simulink model "Simulationsmodell_Diesel"  (R2020b)
settings: Solver=FixedStepAuto  StartTime=0.0  StopTime=simtime  FixedStep=1  RelTol=1e-3
undefined symbols (not defined in the file): c_d, c_r, converter_eff, eta_getriebe, fzBreite, fzBreiteInklSpiegel, fzHoehe, g, i_getriebe, i_mainreducer, kennfeld, lambda, luftdruck, M_bus, M_fahrgast, podesthoehe, R_Reifen, taupunkt, temperatur, torque_outputDivInput, tr_speed_ratio, tr_torque_ratio
settings Model: OrderedModelArguments=off  Creator=igyun  LastModifiedBy=user

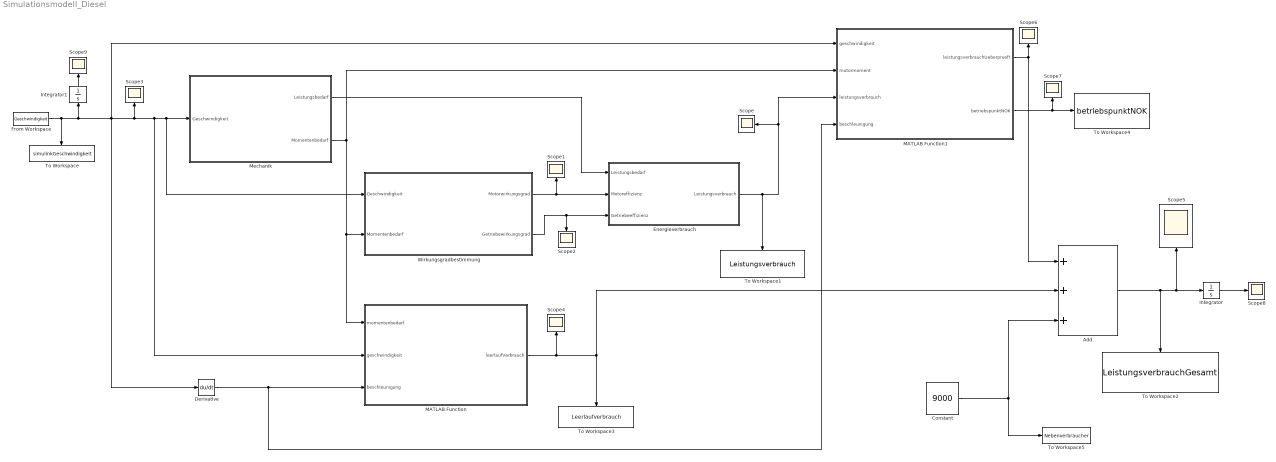
== system Simulationsmodell_Diesel ==
  Add : Sum  Inputs=+++
  Constant : Constant  Value=9000
  Derivative : Derivative
  Energieverbrauch : Subsystem
  From Workspace : FromWorkspace  VariableName=Geschwindigkeit
  Integrator : Integrator
  Integrator1 : Integrator
  MATLAB Function : MATLAB Function  TreatAsAtomicUnit=on
  MATLAB Function1 : MATLAB Function  TreatAsAtomicUnit=on
  Mechanik : Subsystem
  Scope{,1..9} (10 alike) : Scope
  To Workspace : ToWorkspace  VariableName=simulinkGeschwindigkeit  SaveFormat=Timeseries  SampleTime=-1
  To Workspace1 : ToWorkspace  VariableName=Leistungsverbrauch  SaveFormat=Timeseries  SampleTime=-1
  To Workspace2 : ToWorkspace  VariableName=LeistungsverbrauchGesamt  SaveFormat=Timeseries  SampleTime=-1
  To Workspace3 : ToWorkspace  VariableName=Leerlaufverbrauch  SaveFormat=Timeseries  SampleTime=-1
  To Workspace4 : ToWorkspace  VariableName=betriebspunktNOK  SaveFormat=Timeseries  SampleTime=-1
  To Workspace5 : ToWorkspace  VariableName=Nebenverbraucher  SaveFormat=Timeseries  SampleTime=-1
  Wirkungsgradbestimmung : Subsystem
  wires:
  Mechanik/1(Leistungsbedarf) -> Energieverbrauch/1(Leistungsbedarf)
  From Workspace/1 -> Wirkungsgradbestimmung/1(Geschwindigkeit), Mechanik/1(Geschwindigkeit), MATLAB Function/2(geschwindigkeit), Scope3/1, MATLAB Function1/1(geschwindigkeit), Derivative/1, Integrator1/1, To Workspace/1
  Mechanik/2(Momentenbedarf) -> MATLAB Function1/2(motormoment), MATLAB Function/1(momentenbedarf), Wirkungsgradbestimmung/2(Momentenbedarf)
  Wirkungsgradbestimmung/1(Motorwirkungsgrad) -> Scope1/1, Energieverbrauch/2(Motoreffizienz)
  Wirkungsgradbestimmung/2(Getriebewirkungsgrad) -> Energieverbrauch/3(Getriebeeffizienz), Scope2/1
  Energieverbrauch/1(Leistungsverbrauch) -> MATLAB Function1/3(leistungsverbrauch), Scope/1, To Workspace1/1
  Derivative/1 -> MATLAB Function/3(beschleunigung), MATLAB Function1/4(beschleunigung)
  MATLAB Function/1(leerlaufVerbrauch) -> To Workspace3/1, Add/2, Scope4/1
  Add/1 -> To Workspace2/1, Integrator/1, Scope5/1
  MATLAB Function1/1(leistungsverbrauchUeberprueft) -> Add/1, Scope6/1
  MATLAB Function1/2(betriebspunktNOK) -> To Workspace4/1, Scope7/1
  Integrator/1 -> Scope8/1
  Integrator1/1 -> Scope9/1
  Constant/1 -> To Workspace5/1, Add/3

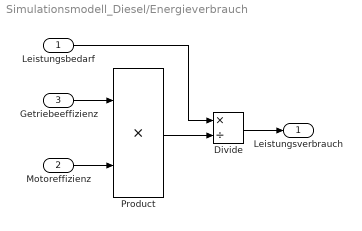
== system Simulationsmodell_Diesel/Energieverbrauch ==
  Leistungsbedarf : Inport
  Motoreffizienz : Inport  Port=2
  Getriebeeffizienz : Inport  Port=3
  Divide : Product  Inputs=*/
  Product : Product
  Leistungsverbrauch : Outport
  wires:
  Getriebeeffizienz/1 -> Product/1
  Motoreffizienz/1 -> Product/2
  Leistungsbedarf/1 -> Divide/1
  Product/1 -> Divide/2
  Divide/1 -> Leistungsverbrauch/1

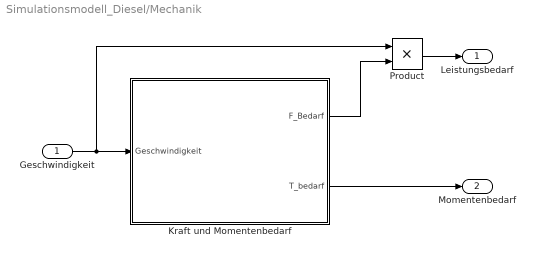
== system Simulationsmodell_Diesel/Mechanik ==
  Geschwindigkeit : Inport
  Kraft und Momentenbedarf : Subsystem
  Product : Product
  Leistungsbedarf : Outport
  Momentenbedarf : Outport  Port=2
  wires:
  Product/1 -> Leistungsbedarf/1
  Kraft und Momentenbedarf/1(F_Bedarf) -> Product/2
  Geschwindigkeit/1 -> Kraft und Momentenbedarf/1(Geschwindigkeit), Product/1
  Kraft und Momentenbedarf/2(T_bedarf) -> Momentenbedarf/1

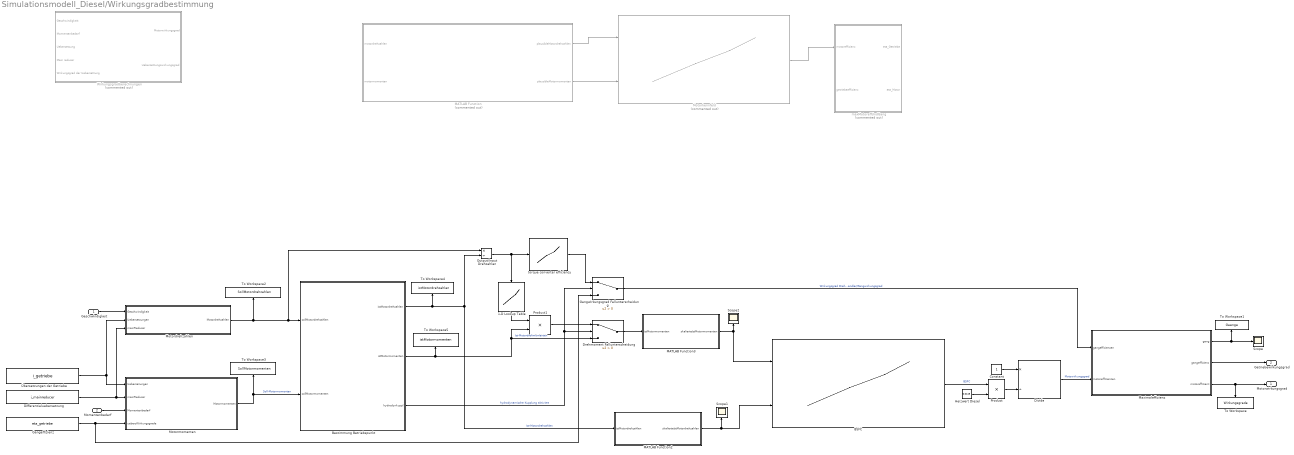
== system Simulationsmodell_Diesel/Wirkungsgradbestimmung ==
  Geschwindigkeit : Inport
  Momentenbedarf : Inport  Port=2
  1-D Lookup Table : Lookup_n-D  NumberOfTableDimensions=1  BreakpointsForDimension1=tr_speed_ratio  Table=tr_torque_ratio  InternalRulePriority=Speed  RndMeth=Simplest  InputSameDT=on
  BSFC : Lookup_n-D  BreakpointsForDimension1=[1:91]  BreakpointsForDimension2=[1:166]  Table=kennfeld  InternalRulePriority=Speed  RndMeth=Simplest  InputSameDT=on
      settings: InputPortMap=u0,u1
  Bestimmung Betriebspunkt : MATLAB Function  TreatAsAtomicUnit=on
  Constant : Constant
  Differentialuebersetzung : Constant  Value=i_mainreducer
  Divide : Product  Inputs=*/
  Drehmoment Fallunterscheidung : Switch  Criteria=u2 > Threshold
  Gangeffizienz : Constant  Value=eta_getriebe
  Gangwirkungsgrad Fallunterscheidung : Switch  Criteria=u2 > Threshold
  Heizwert Diesel : Constant  Value=0.0119
  MATLAB Function : MATLAB Function  Commented=on  TreatAsAtomicUnit=on
  MATLAB Function2 : MATLAB Function  TreatAsAtomicUnit=on
  MATLAB Function3 : MATLAB Function  TreatAsAtomicUnit=on
  Maximaleffizienz : MATLAB Function  TreatAsAtomicUnit=on
  Motordrehzahlen : Subsystem
  Motorkennfeld : Lookup_n-D  Commented=on  BreakpointsForDimension1=[1:86]  BreakpointsForDimension2=[1:251]  Table=kennfeld  InternalRulePriority=Speed  RndMeth=Simplest  InputSameDT=on
      settings: InputPortMap=u0,u1
  Motormomenten : Subsystem
  Output/Input Drehzahlen : Product  Inputs=*/
  Product : Product
  Product1 : Product
  Scope : Scope
  Scope1 : Scope
  Scope2 : Scope
  To Workspace : ToWorkspace  VariableName=Wirkungsgrade  SaveFormat=Timeseries  SampleTime=-1
  To Workspace1 : ToWorkspace  VariableName=Gaenge  SaveFormat=Timeseries  SampleTime=-1
  To Workspace2 : ToWorkspace  VariableName=SollMotordrehzahlen  SaveFormat=Timeseries  SampleTime=-1
  To Workspace3 : ToWorkspace  VariableName=SollMotormomenten  SaveFormat=Timeseries  SampleTime=-1
  To Workspace4 : ToWorkspace  VariableName=istMotordrehzahlen  SaveFormat=Timeseries  SampleTime=-1
  To Workspace5 : ToWorkspace  VariableName=istMotormomenten  SaveFormat=Timeseries  SampleTime=-1
  Wirkungsgradberechnungen : Subsystem  Commented=on  TreatAsAtomicUnit=on
  maxMotoreffUndGang : MATLAB Function  Commented=on  TreatAsAtomicUnit=on
  torque converter efficiency : Lookup_n-D  NumberOfTableDimensions=1  BreakpointsForDimension1=torque_outputDivInput  Table=converter_eff  InternalRulePriority=Speed  RndMeth=Simplest  InputSameDT=on
  Übersetzungen der Getriebe : Constant  Value=i_getriebe
  Motorwirkungsgrad : Outport
  Getriebewirkungsgrad : Outport  Port=2
  wires:
  Übersetzungen der Getriebe/1 -> Motormomenten/1(Uebersezungen), Motordrehzahlen/2(Uebersetzungen)
  Differentialuebersetzung/1 -> Motordrehzahlen/3(mainReducer), Motormomenten/2(mainReducer)
  Momentenbedarf/1 -> Motormomenten/3(Momentenbedarf)
  Gangeffizienz/1 -> Gangwirkungsgrad Fallunterscheidung/3, Motormomenten/4(uebersWirkungsgrade)
  MATLAB Function/1(plausibleMotordrehzahlen) -> Motorkennfeld/1
  MATLAB Function/2(plausibleMotormomenten) -> Motorkennfeld/2
  Motorkennfeld/1 -> maxMotoreffUndGang/1(motoreffizienz)
  Motordrehzahlen/1(Motordrehzahlen) -> To Workspace2/1, Output/Input Drehzahlen/1, Bestimmung Betriebspunkt/1(sollMotordrehzahlen)
  Motormomenten/1(Motormomenten) -> Bestimmung Betriebspunkt/2(sollMotormomenten), To Workspace3/1  "Soll-Motormomenten"
  Bestimmung Betriebspunkt/1(istMotordrehzahlen) -> MATLAB Function2/1(istMotordrehzahlen), Output/Input Drehzahlen/2, To Workspace4/1  "Ist-Motordrehzahlen"
  Output/Input Drehzahlen/1 -> 1-D Lookup Table/1, torque converter efficiency/1
  torque converter efficiency/1 -> Gangwirkungsgrad Fallunterscheidung/1
  Bestimmung Betriebspunkt/2(istMotormomenten) -> Product1/2, Drehmoment Fallunterscheidung/3, To Workspace5/1  "Ist-Motordrehmomenten"
  Bestimmung Betriebspunkt/3(hydrodynkuppl) -> Gangwirkungsgrad Fallunterscheidung/2, Drehmoment Fallunterscheidung/2  "hydrodynamische Kupplung aktiviert"
  Gangwirkungsgrad Fallunterscheidung/1 -> Maximaleffizienz/1(gangeffizienzen)  "Wirkungsgrad Drehmomentwandler/Gangwirkungsgrad"
  Maximaleffizienz/2(gangeffizienz) -> Getriebewirkungsgrad/1
  Maximaleffizienz/3(motoreffizienz) -> Motorwirkungsgrad/1, To Workspace/1
  Maximaleffizienz/1(gang) -> To Workspace1/1, Scope/1
  BSFC/1 -> Product/1  "BSFC"
  Constant/1 -> Divide/1
  Divide/1 -> Maximaleffizienz/2(motoreffizienzen)  "Motowirkungsgrad"
  Heizwert Diesel/1 -> Product/2
  Product/1 -> Divide/2
  1-D Lookup Table/1 -> Product1/1
  Product1/1 -> Drehmoment Fallunterscheidung/1
  Drehmoment Fallunterscheidung/1 -> MATLAB Function3/1(istMotormomenten)
  Geschwindigkeit/1 -> Motordrehzahlen/1(Geschwindigkeit)
  MATLAB Function2/1(skalierteIstMotordrehzahlen) -> BSFC/2, Scope1/1
  MATLAB Function3/1(skalierteIstMotormomenten) -> BSFC/1, Scope2/1

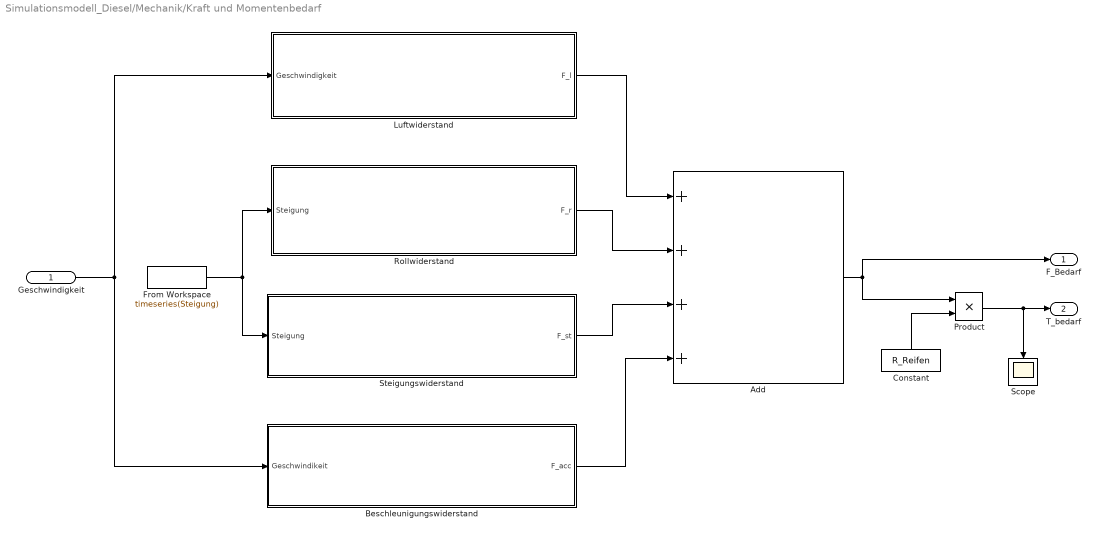
== system Simulationsmodell_Diesel/Mechanik/Kraft und Momentenbedarf ==
  Geschwindigkeit : Inport
  Add : Sum  Inputs=++++
  Beschleunigungswiderstand : Subsystem
  Constant : Constant  Value=R_Reifen
  From Workspace : FromWorkspace  VariableName=timeseries(Steigung)
  Luftwiderstand : Subsystem
  Product : Product
  Rollwiderstand : Subsystem
  Scope : Scope
  Steigungswiderstand : Subsystem
  F_Bedarf : Outport
  T_bedarf : Outport  Port=2
  wires:
  Geschwindigkeit/1 -> Beschleunigungswiderstand/1(Geschwindikeit), Luftwiderstand/1(Geschwindigkeit)
  Luftwiderstand/1(F_l) -> Add/1
  Beschleunigungswiderstand/1(F_acc) -> Add/4
  Rollwiderstand/1(F_r) -> Add/2
  Steigungswiderstand/1(F_st) -> Add/3
  Add/1 -> Product/1, F_Bedarf/1
  Constant/1 -> Product/2
  Product/1 -> T_bedarf/1, Scope/1
  From Workspace/1 -> Steigungswiderstand/1(Steigung), Rollwiderstand/1(Steigung)

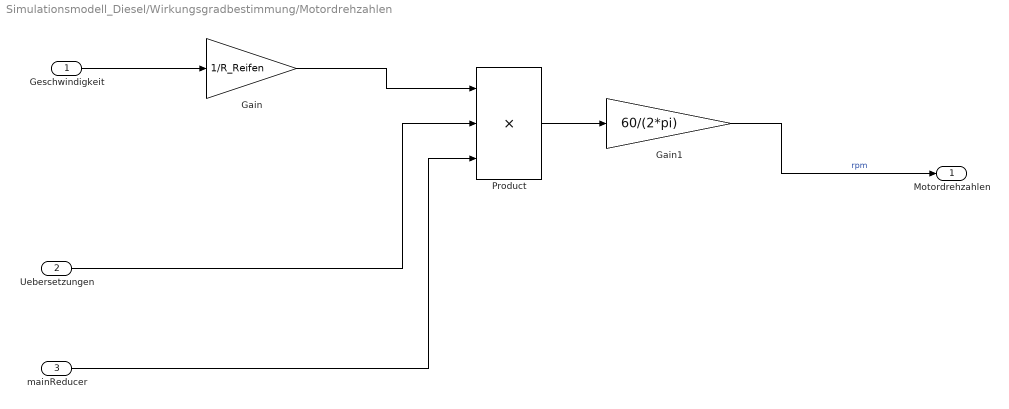
== system Simulationsmodell_Diesel/Wirkungsgradbestimmung/Motordrehzahlen ==
  Geschwindigkeit : Inport
  Uebersetzungen : Inport  Port=2
  mainReducer : Inport  Port=3
  Gain : Gain  Gain=1/R_Reifen
  Gain1 : Gain  Gain=60/(2*pi)
  Product : Product  Inputs=3
  Motordrehzahlen : Outport
  wires:
  Geschwindigkeit/1 -> Gain/1
  Product/1 -> Gain1/1
  Uebersetzungen/1 -> Product/2
  Gain/1 -> Product/1
  mainReducer/1 -> Product/3
  Gain1/1 -> Motordrehzahlen/1  "rpm"

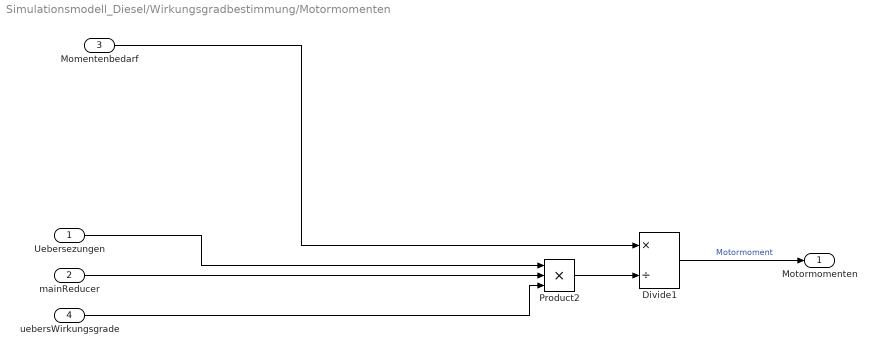
== system Simulationsmodell_Diesel/Wirkungsgradbestimmung/Motormomenten ==
  Uebersezungen : Inport
  mainReducer : Inport  Port=2
  Momentenbedarf : Inport  Port=3
  uebersWirkungsgrade : Inport  Port=4
  Divide1 : Product  Inputs=*/
  Product2 : Product  Inputs=3
  Motormomenten : Outport
  wires:
  uebersWirkungsgrade/1 -> Product2/3
  mainReducer/1 -> Product2/2
  Product2/1 -> Divide1/2
  Momentenbedarf/1 -> Divide1/1
  Uebersezungen/1 -> Product2/1
  Divide1/1 -> Motormomenten/1  "Motormoment"

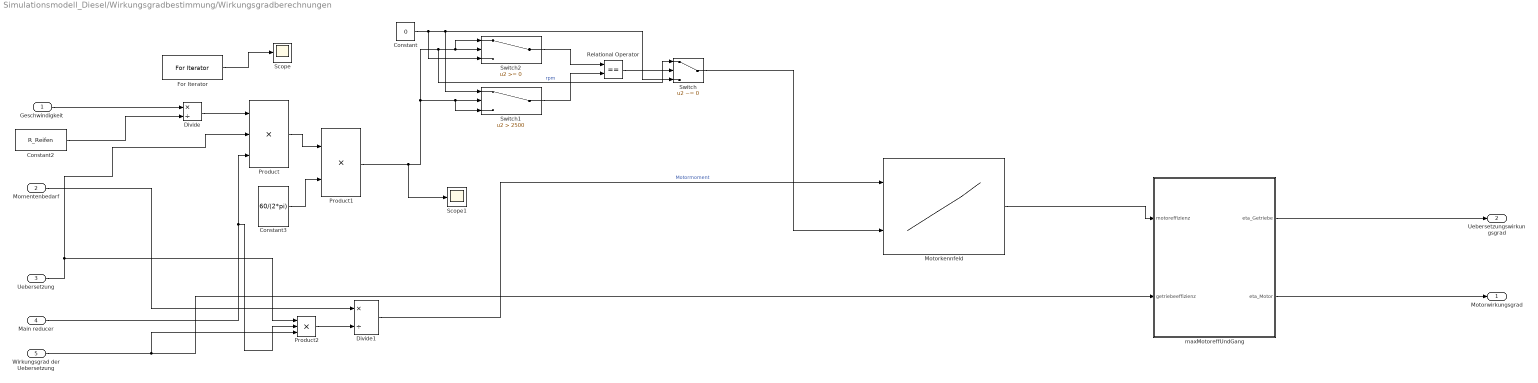
== system Simulationsmodell_Diesel/Wirkungsgradbestimmung/Wirkungsgradberechnungen ==
  Geschwindigkeit : Inport
  Momentenbedarf : Inport  Port=2
  Uebersetzung : Inport  Port=3
  Main reducer : Inport  Port=4
  Wirkungsgrad der Uebersetzung : Inport  Port=5
  Constant : Constant  Value=0
  Constant2 : Constant  Value=R_Reifen
  Constant3 : Constant  Value=60/(2*pi)
  Divide : Product  Inputs=*/
  Divide1 : Product  Inputs=*/
  For Iterator : ForIterator  IterationLimit=4
  Motorkennfeld : Lookup_n-D  BreakpointsForDimension1=[1:86]  BreakpointsForDimension2=[1:251]  Table=kennfeld  InternalRulePriority=Speed  RndMeth=Simplest  InputSameDT=on
      settings: InputPortMap=u0,u1
  Product : Product  Inputs=3
  Product1 : Product
  Product2 : Product  Inputs=3
  Relational Operator : RelationalOperator  Operator===  OutDataTypeStr=boolean  RndMeth=Simplest
  Scope : Scope
  Scope1 : Scope
  Switch : Switch  Criteria=u2 ~= 0  Threshold=1
  Switch1 : Switch  Criteria=u2 > Threshold  Threshold=2500
  Switch2 : Switch
  maxMotoreffUndGang : MATLAB Function  TreatAsAtomicUnit=on
  Motorwirkungsgrad : Outport
  Uebersetzungswirkungsgrad : Outport  Port=2
  wires:
  Constant3/1 -> Product1/2
  Product/1 -> Product1/1
  Constant2/1 -> Divide/2
  Geschwindigkeit/1 -> Divide/1
  Divide/1 -> Product/1
  Wirkungsgrad der Uebersetzung/1 -> maxMotoreffUndGang/2(getriebeeffizienz), Product2/3
  Main reducer/1 -> Product2/2, Product/3
  Uebersetzung/1 -> Product/2, Product2/1
  Product2/1 -> Divide1/2
  Momentenbedarf/1 -> Divide1/1
  Divide1/1 -> Motorkennfeld/1  "Motormoment"
  Motorkennfeld/1 -> maxMotoreffUndGang/1(motoreffizienz)
  maxMotoreffUndGang/1(eta_Getriebe) -> Uebersetzungswirkungsgrad/1
  maxMotoreffUndGang/2(eta_Motor) -> Motorwirkungsgrad/1
  For Iterator/1 -> Scope/1
  Switch2/1 -> Relational Operator/1
  Switch1/1 -> Relational Operator/2
  Constant/1 -> Switch2/3, Switch1/1, Switch/3
  Switch/1 -> Motorkennfeld/2
  Relational Operator/1 -> Switch/2
  Product1/1 -> Scope1/1, Switch1/3, Switch1/2, Switch/1, Switch2/1, Switch2/2  "rpm"

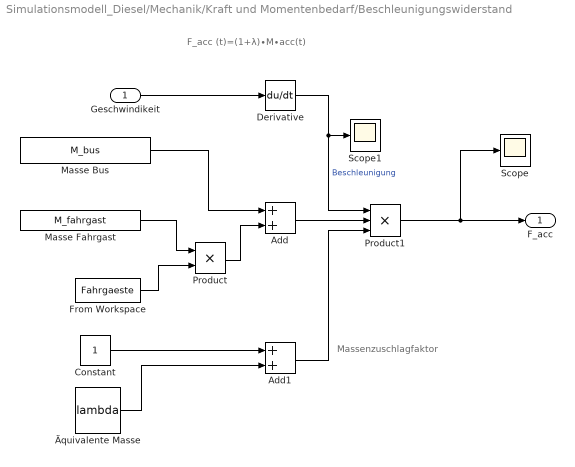
== system Simulationsmodell_Diesel/Mechanik/Kraft und Momentenbedarf/Beschleunigungswiderstand ==
  note: Massenzuschlagfaktor
  note: F_acc (t)=(1+λ)∙M∙acc(t)
  Geschwindikeit : Inport
  Add : Sum
  Add1 : Sum
  Constant : Constant
  Derivative : Derivative
  From Workspace : FromWorkspace  VariableName=Fahrgaeste
  Masse Bus : Constant  Value=M_bus
  Masse Fahrgast : Constant  Value=M_fahrgast
  Product : Product
  Product1 : Product  Inputs=3
  Scope : Scope
  Scope1 : Scope
  Äquivalente Masse : Constant  Value=lambda
  F_acc : Outport
  wires:
  Geschwindikeit/1 -> Derivative/1
  Masse Fahrgast/1 -> Product/1
  From Workspace/1 -> Product/2
  Masse Bus/1 -> Add/1
  Product/1 -> Add/2
  Constant/1 -> Add1/1
  Äquivalente Masse/1 -> Add1/2
  Derivative/1 -> Product1/1, Scope1/1  "Beschleunigung"
  Add/1 -> Product1/2
  Add1/1 -> Product1/3
  Product1/1 -> Scope/1, F_acc/1

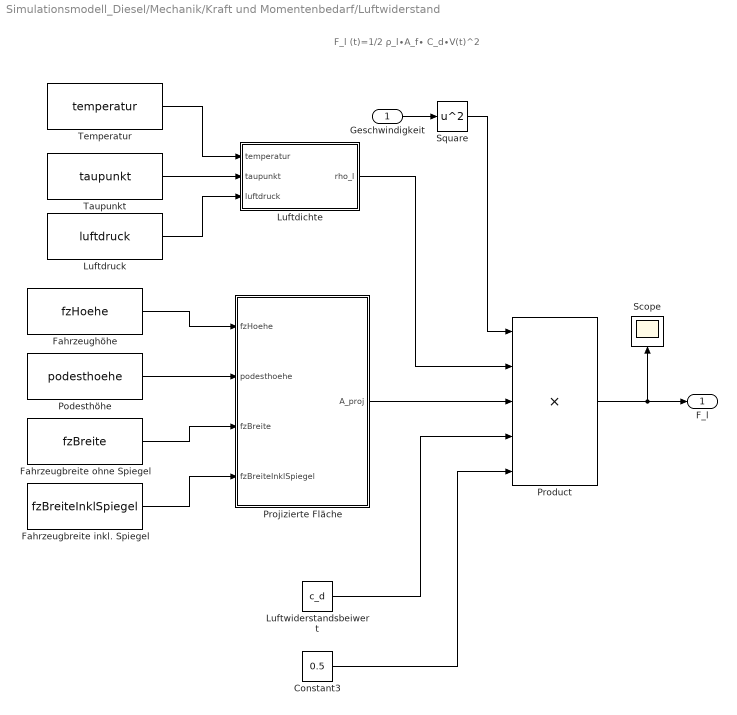
== system Simulationsmodell_Diesel/Mechanik/Kraft und Momentenbedarf/Luftwiderstand ==
  note: F_l (t)=1/2 ρ_l∙A_f∙ C_d∙V(t)^2
  Geschwindigkeit : Inport
  Constant3 : Constant  Value=0.5
  Fahrzeugbreite inkl. Spiegel : Constant  Value=fzBreiteInklSpiegel
  Fahrzeugbreite ohne Spiegel : Constant  Value=fzBreite
  Fahrzeughöhe : Constant  Value=fzHoehe
  Luftdichte : MATLAB Function  TreatAsAtomicUnit=on
  Luftdruck : Constant  Value=luftdruck
  Luftwiderstandsbeiwert : Constant  Value=c_d
  Podesthöhe : Constant  Value=podesthoehe
  Product : Product  Inputs=5
  Projizierte Fläche : MATLAB Function  TreatAsAtomicUnit=on
  Scope : Scope
  Square : Math  Operator=square  SaturateOnIntegerOverflow=on
  Taupunkt : Constant  Value=taupunkt
  Temperatur : Constant  Value=temperatur
  F_l : Outport
  wires:
  Geschwindigkeit/1 -> Square/1
  Square/1 -> Product/1
  Luftdichte/1(rho_l) -> Product/2
  Projizierte Fläche/1(A_proj) -> Product/3
  Luftwiderstandsbeiwert/1 -> Product/4
  Constant3/1 -> Product/5
  Product/1 -> F_l/1, Scope/1
  Temperatur/1 -> Luftdichte/1(temperatur)
  Taupunkt/1 -> Luftdichte/2(taupunkt)
  Luftdruck/1 -> Luftdichte/3(luftdruck)
  Fahrzeugbreite inkl. Spiegel/1 -> Projizierte Fläche/4(fzBreiteInklSpiegel)
  Fahrzeugbreite ohne Spiegel/1 -> Projizierte Fläche/3(fzBreite)
  Podesthöhe/1 -> Projizierte Fläche/2(podesthoehe)
  Fahrzeughöhe/1 -> Projizierte Fläche/1(fzHoehe)

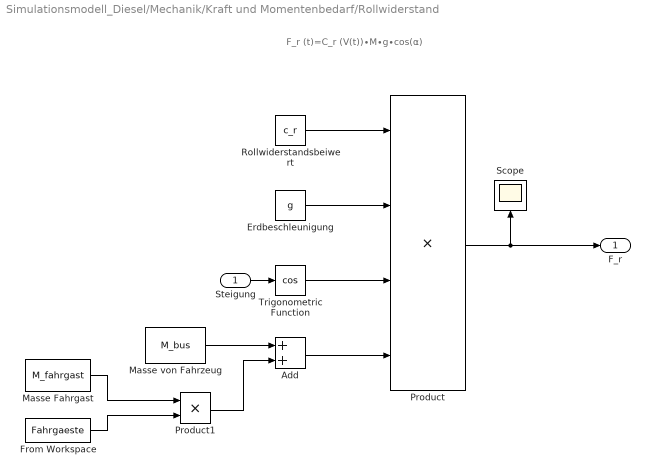
== system Simulationsmodell_Diesel/Mechanik/Kraft und Momentenbedarf/Rollwiderstand ==
  note: F_r (t)=C_r (V(t))∙M∙g∙cos⁡(α)
  Steigung : Inport
  Add : Sum
  Erdbeschleunigung : Constant  Value=g
  From Workspace : FromWorkspace  VariableName=Fahrgaeste
  Masse Fahrgast : Constant  Value=M_fahrgast
  Masse von Fahrzeug : Constant  Value=M_bus
  Product : Product  Inputs=4
  Product1 : Product
  Rollwiderstandsbeiwert : Constant  Value=c_r
  Scope : Scope
  Trigonometric Function : Trigonometry  Operator=cos
  F_r : Outport
  wires:
  Masse von Fahrzeug/1 -> Add/1
  Steigung/1 -> Trigonometric Function/1
  Add/1 -> Product/4
  Trigonometric Function/1 -> Product/3
  Erdbeschleunigung/1 -> Product/2
  Rollwiderstandsbeiwert/1 -> Product/1
  Product/1 -> F_r/1, Scope/1
  Masse Fahrgast/1 -> Product1/1
  From Workspace/1 -> Product1/2
  Product1/1 -> Add/2

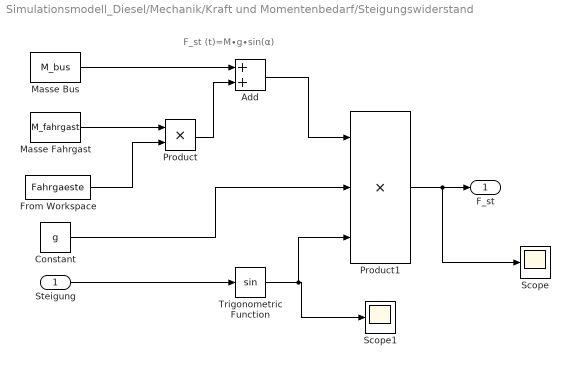
== system Simulationsmodell_Diesel/Mechanik/Kraft und Momentenbedarf/Steigungswiderstand ==
  note: F_st (t)=M∙g∙sin⁡(α)
  Steigung : Inport
  Add : Sum
  Constant : Constant  Value=g
  From Workspace : FromWorkspace  VariableName=Fahrgaeste
  Masse Bus : Constant  Value=M_bus
  Masse Fahrgast : Constant  Value=M_fahrgast
  Product : Product
  Product1 : Product  Inputs=3
  Scope : Scope
  Scope1 : Scope
  Trigonometric Function : Trigonometry
  F_st : Outport
  wires:
  Masse Fahrgast/1 -> Product/1
  From Workspace/1 -> Product/2
  Masse Bus/1 -> Add/1
  Product/1 -> Add/2
  Steigung/1 -> Trigonometric Function/1
  Add/1 -> Product1/1
  Trigonometric Function/1 -> Product1/3, Scope1/1
  Product1/1 -> Scope/1, F_st/1
  Constant/1 -> Product1/2

== matlab function Simulationsmodell_Diesel/MATLAB Function1 ==
  data: geschwindigkeit input; motormoment input; leistungsverbrauch input; leistungsverbrauchUeberprueft output; beschleunigung input; betriebspunktNOK output
function [leistungsverbrauchUeberprueft, betriebspunktNOK] = ueberpruefeNaN(geschwindigkeit, motormoment, leistungsverbrauch, beschleunigung)

    if isnan(leistungsverbrauch)
        if (geschwindigkeit == 0 && beschleunigung == 0) || motormoment <= 0
            leistungsverbrauchUeberprueft = 0;
            betriebspunktNOK = 0;
        else
            betriebspunktNOK = 1;
            leistungsverbrauchUeberprueft = 0;
        end
    else
        betriebspunktNOK = 0;
        leistungsverbrauchUeberprueft = leistungsverbrauch;
    end
        


end

== matlab function Simulationsmodell_Diesel/Mechanik/Kraft und Momentenbedarf/Luftwiderstand/Projizierte Fläche ==
  data: fzHoehe input; A_proj output; podesthoehe input; fzBreite input; fzBreiteInklSpiegel input
function A_proj = projflaeche(fzHoehe, podesthoehe, fzBreite, fzBreiteInklSpiegel)

    %Eingabe in Maske: mm
    
    A_proj1 = (fzHoehe-podesthoehe)*fzBreite;
    
    %Spiegelhöhe
    spiegelHoehe = 400;
    A_proj2 = (fzBreiteInklSpiegel-fzBreite)*spiegelHoehe;
    
    A_proj = A_proj1 + A_proj2;
    
    %Umrechung mm^2 in m^2;
    
    A_proj = A_proj * 10^-6;
    
end

== matlab function Simulationsmodell_Diesel/Mechanik/Kraft und Momentenbedarf/Luftwiderstand/Luftdichte ==
  data: temperatur input; rho_l output; taupunkt input; luftdruck input
function rho_l = luftdichte(temperatur, taupunkt, luftdruck)

%Für Werte: https://kachelmannwetter.com/site/auswahl

%Einheiten bei der Eingabemaske:
%Druck: hPa
%Temperatur: Celsius

%Temperaturumrechnung
temperatur = temperatur + 273.15;



%Konstanten aus https://www.gribble.org/cycling/air_density.html
c0 = 0.99999683;
c1 = -0.90826951e-2;
c2 = 0.78736169e-4;
c3 = -0.61117958e-6;
c4 = 0.43884187e-8;
c5 = -0.29883885e-10;
c6 = 0.21874425e-12;
c7 = -0.17892321e-14;
c8 = 0.11112018e-16;
c9 = -0.30994571e-19;

e_so = 6.1078;

R_v = 461.4964;
R_d=287.0531;

%Druck bei Sättigungstemperatur
p_taupunkt = c0 + taupunkt *(c1 + taupunkt*(c2 + taupunkt*(c3 + taupunkt*(c4 + taupunkt*(c5 + taupunkt*(c6 + taupunkt*(c7 + taupunkt*(c8 + taupunkt*(c9) ) ) ) ) ) ) ));

%Sättigungsdruck von Dampf
E_s = e_so./p_taupunkt.^8;
P_v = E_s;

%Luftdruck bei trockener Luft
P_d = luftdruck - P_v;

%Luftdichte in kg/m^3
rho_l =  (P_d*100 / (R_d * temperatur)) + (P_v*100 / (R_v * temperatur));
%Umrechnungsfaktor 100 von mbar(hPa) zu Pa
end

== matlab function Simulationsmodell_Diesel/Wirkungsgradbestimmung/MATLAB Function ==
  data: motordrehzahlen input; plausibleMotordrehzahlen output; motormomenten input; plausibleMotormomenten output
function [plausibleMotordrehzahlen, plausibleMotormomenten] = ueberpruefenDrehzahlDrehmoment(motordrehzahlen, motormomenten)
    %Vorerzeugen der Vektoren mit plausiblen Daten
    plausibleMotordrehzahlen = zeros(4,1);
    plausibleMotormomenten = zeros(4,1);
    for j = 1:4 %4 Gänge => 4 drehzahlen bzw. momenten
        if motordrehzahlen(j)<=2500 && motordrehzahlen(j)>=800 && motormomenten(j)>=0 && motormomenten(j)<=1200
            %Wenn die Bedingungen erfüllt sind, ist der Betriebspunkt
            %erreichbar
            plausibleMotordrehzahlen(j,1)=motordrehzahlen(j);
            plausibleMotormomenten(j,1)=motormomenten(j);
        else
            plausibleMotordrehzahlen(j,1)=0;
            plausibleMotormomenten(j,1)=0;
        end
    end
end

== matlab function Simulationsmodell_Diesel/Wirkungsgradbestimmung/Wirkungsgradberechnungen/maxMotoreffUndGang ==
  data: motoreffizienz input; eta_Getriebe output; getriebeeffizienz input; eta_Motor output
function [eta_Getriebe, eta_Motor] = wirkungsgradAuswahl(motoreffizienz, getriebeeffizienz)

for j = 2:length(motoreffizienz)
    if motoreffizienz(j)>motoreffizienz(j-1)
        index = j;
    else
        index = j-1;
    end
end
eta_Getriebe = getriebeeffizienz(index);
eta_Motor = motoreffizienz(index);

== matlab function Simulationsmodell_Diesel/Wirkungsgradbestimmung/maxMotoreffUndGang ==
  data: motoreffizienz input; eta_Getriebe output; getriebeeffizienz input; eta_Motor output
function [eta_Getriebe, eta_Motor] = wirkungsgradAuswahl(motoreffizienz, getriebeeffizienz)

for j = 2:length(motoreffizienz)
    if motoreffizienz(j)>motoreffizienz(j-1)
        index = j;
    else
        index = j-1;
    end
end
eta_Getriebe = getriebeeffizienz(index);
eta_Motor = motoreffizienz(index);

== matlab function Simulationsmodell_Diesel/Wirkungsgradbestimmung/Bestimmung Betriebspunkt ==
  data: sollMotordrehzahlen input; istMotordrehzahlen output; istMotormomenten output; hydrodynkuppl output; sollMotormomenten input
function [istMotordrehzahlen, istMotormomenten, hydrodynkuppl]  = betriebspunktBestimmungen(sollMotordrehzahlen, sollMotormomenten)
    
    %Mindestdrehzahlbestimmung 
    
    if sollMotordrehzahlen(1) < 800
        istMotordrehzahlen = zeros(length(sollMotordrehzahlen),1);
        %Für den Fall, dass sogar erster Gang die notwendige
        %Motordrehzahl nicht erreichen kann
        %Annahme: Minimaldrehzahl = 800 rpm
        
        istMotordrehzahlen(1) = 800; 
        
        %Hilfsvariable (es handelt sich um eine hydrodynamische Kupplung)
        hydrodynkuppl = 1;
        
        %Die restlichen Motordrehzahlen als NaN definieren
        
        istMotordrehzahlen(2) = NaN;
        istMotordrehzahlen(3) = NaN;
        istMotordrehzahlen(4) = NaN;
    else
        %Die notwendige Drehzahl wird mindestens von 1. Gang erreicht =>
        %keine hydrodynamische Kupplung notwendig
        hydrodynkuppl = 0;
        
        %Vorerzeugung der Größe des Vektors
        
        istMotordrehzahlen=zeros(length(sollMotordrehzahlen),1);
        
        %Überprüfen ob die Gänge im zul. Bereich liegen

        for ii = 1:length(sollMotordrehzahlen)
            if sollMotordrehzahlen(ii) >= 800 && sollMotordrehzahlen(ii) <= 2500
                %Zuvor berechnete Werte (soll) liegen im zul. Bereich =>
                %ist=soll
                istMotordrehzahlen(ii)=sollMotordrehzahlen(ii);
            else
                istMotordrehzahlen(ii) = NaN;
            end
        end
    end
    
    %zul. Drehmomente
    istMotormomenten = zeros(length(sollMotormomenten),1);
    
    for ii = 1:length(sollMotormomenten)
        
        %Definition der Obergrenze
        if sollMotormomenten(ii) >= 0 && sollMotormomenten(ii) <= 1200
            istMotormomenten(ii) = sollMotormomenten(ii);
        else
            istMotormomenten(ii) = NaN;
        end
        
    end


    
end

== matlab function Simulationsmodell_Diesel/Wirkungsgradbestimmung/Maximaleffizienz ==
  data: gang output; gangeffizienzen input; motoreffizienzen input; gangeffizienz output; motoreffizienz output
function [gang, gangeffizienz, motoreffizienz]= maxEff(gangeffizienzen, motoreffizienzen)

    %Für die ermittelten Motoreffizienzen (bei 4 Gänge => 4) wird das
    %Maximum bestimmt. Außerdem wird der zugehörige Gang ermittelt und der
    %entsprechende Wirkungsgrad
    
    [motoreffizienz, maxIndex] = max(motoreffizienzen);
    
    gang = maxIndex;
    gangeffizienz = gangeffizienzen(maxIndex);
    

end

== matlab function Simulationsmodell_Diesel/Wirkungsgradbestimmung/MATLAB Function3 ==
  data: istMotormomenten input; skalierteIstMotormomenten output
function skalierteIstMotormomenten = skalierungMoment(istMotormomenten)

    %Motormomentbereich des verwendeten Kennfelds 
    %torqueBereichKennfeld = [minKennfeldTorque; maxKennfeldTorque]
    %Einheit: Nm
    %----------!!!Anpassungsbedarf!!!-----------
    minKennfeldTorque = 1;
    maxKennfeldTorque = 91;
    
    torqueBereichKennfeld = maxKennfeldTorque - minKennfeldTorque;
    
    
    %Motormomentbereich des Motors
    %torqueBereichMotor = [minMotorTorque, maxMotorTorque]
    %Einheit Nm
    minMotorTorque = 0;
    maxMotorTorque = 1200;
    
    torqueBereichMotor = maxMotorTorque - minMotorTorque;
    
    %Formel
    skalierteIstMotormomenten = minKennfeldTorque + (torqueBereichKennfeld/torqueBereichMotor)*(istMotormomenten-minMotorTorque);

end

== matlab function Simulationsmodell_Diesel/Wirkungsgradbestimmung/MATLAB Function2 ==
  data: istMotordrehzahlen input; skalierteIstMotordrehzahlen output
function skalierteIstMotordrehzahlen  = skalierungDrehzahl(istMotordrehzahlen)

    %Drehzahlenbereich des verwendeten Kennfelds 
    %rpmBereichKennfeld = [minKennfeldRPM; maxKennfeldRPM]
    %Einheit: U/min
    %----------!!!Anpassungsbedarf!!!-----------
    minKennfeldRPM = 1;
    maxKennfeldRPM = 166;
    
    rpmBereichKennfeld = maxKennfeldRPM - minKennfeldRPM;
    
    
    %Drehzahlenbereich des Motors
    %rpmBereichMotor = [minMotorRPM, maxMotorRPM]
    %Einheit U/min
    minMotorRPM = 800;
    maxMotorRPM = 2500;
    
    rpmBereichMotor = maxMotorRPM - minMotorRPM;
    
    %Formel
    skalierteIstMotordrehzahlen = minKennfeldRPM + (rpmBereichKennfeld/rpmBereichMotor)*(istMotordrehzahlen-minMotorRPM);
end

== matlab function Simulationsmodell_Diesel/MATLAB Function ==
  data: momentenbedarf input; geschwindigkeit input; leerlaufVerbrauch output; beschleunigung input
function leerlaufVerbrauch = leerlaufVerbrauch(momentenbedarf,geschwindigkeit, beschleunigung)

    if (geschwindigkeit == 0 && beschleunigung == 0) || momentenbedarf <= 0
        leerlaufVerbrauch = 10.71e3;
    else
        leerlaufVerbrauch = 0;
    end

end
